simulink model "task1_simple_model_channels_gaussians"  (R2020b)
settings: Solver=VariableStepAuto  StartTime=0.0  StopTime=20  RelTol=1e-3
libraries: simulink x2, dspsigops x1
settings Model: Creator=Isabel  LastModifiedBy=Isabel

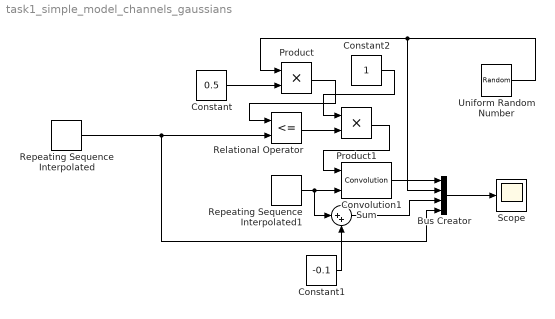
== system task1_simple_model_channels_gaussians ==
  Bus Creator : BusCreator  Inputs=4
  Constant : Constant  Value=0.5
  Constant1 : Constant  Value=-0.1
  Constant2 : Constant
  Convolution1 : dspsigops/Convolution  domain=Time  roundingMode=Floor  overflowMode=off  outputDataTypeStr=Inherit: Same as accumulator  outputMin=[]  outputMax=[]  outputLastDataTypeStr=Inherit: Same as accumulator
      settings: SourceProductBaseCode=DS
  Product : Product
  Product1 : Product
  Relational Operator : RelationalOperator  Operator=<=  OutDataTypeStr=boolean  RndMeth=Simplest
  Repeating Sequence Interpolated : simulink/Sources/Repeating Sequence Interpolated  OutValues=[0 0.027 0.15 0.364 0.49 0.52 0.513 0.489 0.277 0.233 0.18 0.074 0.0177 0 0].'  TimeValues=[0 0.7 1.2 1.6 1.9 2.1 2.2 2.3 2.9 3.1 3.5 4.4 5.2 6.4 8].'  LookUpMeth=Interpolation-Use End Values  tsamp=0.1  OutMin=[]  OutMax=[]  OutDataTypeStr=double  OutputDataTypeScalingMode=double  OutDataType=fixdt(0,8)  OutScaling=2^-10
  Repeating Sequence Interpolated1 : simulink/Sources/Repeating Sequence Interpolated  OutValues=[0.005 0.01 0.018 0.021 0.033 0.053 0.048 0.028 0.01 0.002 0 0].'  TimeValues=[0 0.0015 0.0035 0.004 0.006 0.01 0.014 0.018 0.02 0.026 0.033 0.05].'  LookUpMeth=Interpolation-Use End Values  tsamp=0.0005  OutMin=[]  OutMax=[]  OutDataTypeStr=double  OutputDataTypeScalingMode=double  OutDataType=fixdt(0,8)  OutScaling=2^-10
  Scope : Scope
  Sum : Sum  Inputs=|++
  Uniform Random Number : UniformRandomNumber  Minimum=0  SampleTime=0.1
  wires:
  Uniform Random Number/1 -> Bus Creator/2, Product/1
  Product/1 -> Relational Operator/1
  Bus Creator/1 -> Scope/1
  Repeating Sequence Interpolated/1 -> Bus Creator/4, Relational Operator/2
  Convolution1/1 -> Bus Creator/1
  Repeating Sequence Interpolated1/1 -> Sum/1, Convolution1/2
  Relational Operator/1 -> Product1/2
  Product1/1 -> Convolution1/1
  Constant2/1 -> Product1/1
  Constant/1 -> Product/2
  Constant1/1 -> Sum/2
  Sum/1 -> Bus Creator/3
